simulink library "escontroller_lib"  (R2024a)
settings: Solver=VariableStepAuto  StartTime=0.0  StopTime=10.0  RelTol=1e-3
undefined symbols (not defined in the file): DiscIntNeverNeededParam, theta0
settings Model: Creator=tn212  LastModifiedBy=tn212

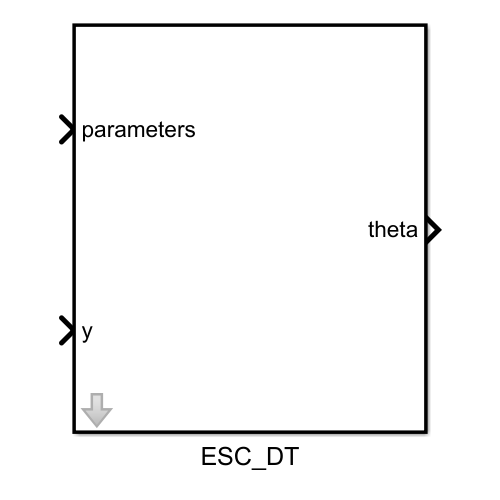
[thumbnail: Simulink's stored preview of the top-level diagram]
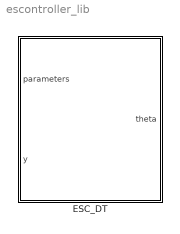
== system escontroller_lib ==
  ESC_DT : Subsystem  TreatAsAtomicUnit=on  mask{offset_sinwave_modulation=0, offset_sinwave_demodulation=0}
      mask prompts: offset_sinwave_modulation "Modulation Sine Wave Offset"; offset_sinwave_demodulation "Demodulation Sine Wave Offset"

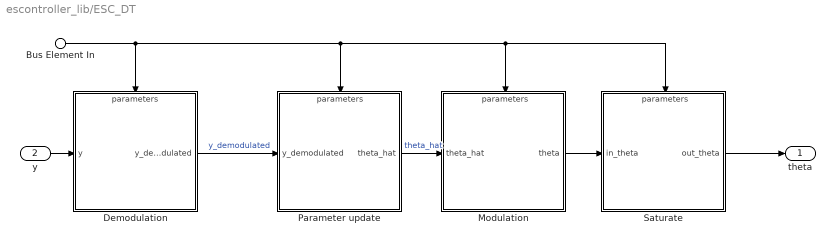
== system escontroller_lib/ESC_DT ==
  Bus Element In : Inport  PortName=parameters
  y : Inport  Port=2
  Demodulation : Subsystem
      settings: PortSchema="{\"entries\":[{\"content\":{\"sides\":[{\"content\":{\"connectorIds\":[\"In1\"]},\"type\":\"ConnectorPlacement.EquallySpacedRectSide\",\"uuid\":\"9be20e08-1b04-4097-90e8-af3e7d9708a2\"},{\"content\":{\"connectorIds\":[\"Out1\"],\"side\":\"RIGHT\"},\"type\":\"ConnectorPlacement.EquallySpacedRectSide\",\"uuid\":\"f95c4cce-30aa-41a8-9527-7dbc7585a088\"},{\"content\":{\"connectorIds\":[\"In2\"],\"side\":\"TOP\"},\"type\":\"ConnectorPlacement.EquallySpacedRectSide\",\"uuid\":\"f76abcb4-2537-40d6-8bec-356143dfe4be\"}]},\"type\":\"ConnectorPlacement.EquallySpacedConnector\",\"uuid\":\"d9c63798-3d6c-4302-a506-66d2b025211e\"}],\"packageUris\":[\"http://schema.mathworks.com/mf0/Connector/R2020b\"],\"version\":\"1.0\"}"
  Modulation : Subsystem
      settings: PortSchema="{\"entries\":[{\"content\":{\"sides\":[{\"content\":{\"connectorIds\":[\"In1\"]},\"type\":\"ConnectorPlacement.EquallySpacedRectSide\",\"uuid\":\"9be20e08-1b04-4097-90e8-af3e7d9708a2\"},{\"content\":{\"connectorIds\":[\"Out1\"],\"side\":\"RIGHT\"},\"type\":\"ConnectorPlacement.EquallySpacedRectSide\",\"uuid\":\"f95c4cce-30aa-41a8-9527-7dbc7585a088\"},{\"content\":{\"connectorIds\":[\"In2\"],\"side\":\"TOP\"},\"type\":\"ConnectorPlacement.EquallySpacedRectSide\",\"uuid\":\"f76abcb4-2537-40d6-8bec-356143dfe4be\"}]},\"type\":\"ConnectorPlacement.EquallySpacedConnector\",\"uuid\":\"d9c63798-3d6c-4302-a506-66d2b025211e\"}],\"packageUris\":[\"http://schema.mathworks.com/mf0/Connector/R2020b\"],\"version\":\"1.0\"}"
  Parameter update : Subsystem
      settings: PortSchema="{\"entries\":[{\"content\":{\"sides\":[{\"content\":{\"connectorIds\":[\"In1\"]},\"type\":\"ConnectorPlacement.EquallySpacedRectSide\",\"uuid\":\"9be20e08-1b04-4097-90e8-af3e7d9708a2\"},{\"content\":{\"connectorIds\":[\"Out1\"],\"side\":\"RIGHT\"},\"type\":\"ConnectorPlacement.EquallySpacedRectSide\",\"uuid\":\"f95c4cce-30aa-41a8-9527-7dbc7585a088\"},{\"content\":{\"connectorIds\":[\"In2\"],\"side\":\"TOP\"},\"type\":\"ConnectorPlacement.EquallySpacedRectSide\",\"uuid\":\"f76abcb4-2537-40d6-8bec-356143dfe4be\"}]},\"type\":\"ConnectorPlacement.EquallySpacedConnector\",\"uuid\":\"d9c63798-3d6c-4302-a506-66d2b025211e\"}],\"packageUris\":[\"http://schema.mathworks.com/mf0/Connector/R2020b\"],\"version\":\"1.0\"}"
  Saturate : Subsystem
      settings: PortSchema="{\"entries\":[{\"content\":{\"sides\":[{\"content\":{\"connectorIds\":[\"In1\"]},\"type\":\"ConnectorPlacement.EquallySpacedRectSide\",\"uuid\":\"9be20e08-1b04-4097-90e8-af3e7d9708a2\"},{\"content\":{\"connectorIds\":[\"Out1\"],\"side\":\"RIGHT\"},\"type\":\"ConnectorPlacement.EquallySpacedRectSide\",\"uuid\":\"f95c4cce-30aa-41a8-9527-7dbc7585a088\"},{\"content\":{\"connectorIds\":[\"In2\"],\"side\":\"TOP\"},\"type\":\"ConnectorPlacement.EquallySpacedRectSide\",\"uuid\":\"f76abcb4-2537-40d6-8bec-356143dfe4be\"}]},\"type\":\"ConnectorPlacement.EquallySpacedConnector\",\"uuid\":\"d9c63798-3d6c-4302-a506-66d2b025211e\"}],\"packageUris\":[\"http://schema.mathworks.com/mf0/Connector/R2020b\"],\"version\":\"1.0\"}"
  theta : Outport
  wires:
  Bus Element In/1 -> Demodulation/2(parameters), Parameter update/2(parameters), Saturate/2(parameters), Modulation/2(parameters)
  Saturate/1(out_theta) -> theta/1
  Modulation/1(theta) -> Saturate/1(in_theta)
  Demodulation/1(y_demodulated) -> Parameter update/1(y_demodulated)  "y_demodulated"
  Parameter update/1(theta_hat) -> Modulation/1(theta_hat)  "theta_hat"
  y/1 -> Demodulation/1(y)

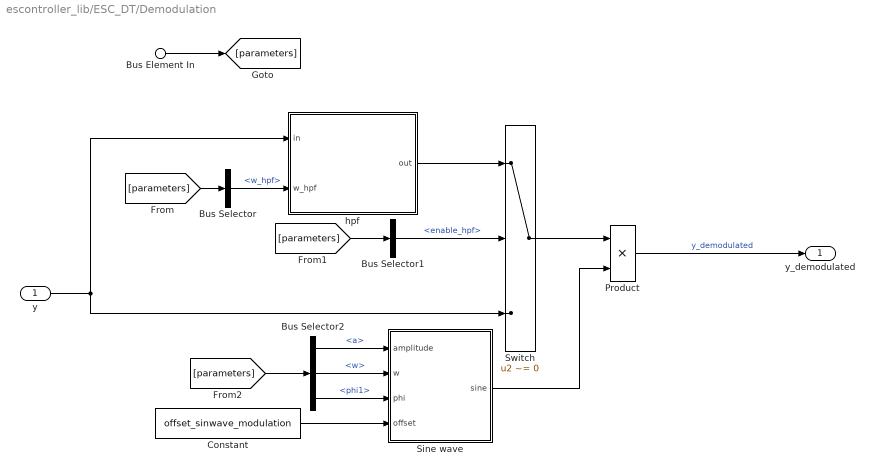
== system escontroller_lib/ESC_DT/Demodulation ==
  y : Inport
  Bus Element In : Inport  Port=2  PortName=parameters
  Bus Selector : BusSelector  OutputSignals=w_hpf
  Bus Selector1 : BusSelector  OutputSignals=enable_hpf
  Bus Selector2 : BusSelector  OutputSignals=a,w,phi1
  Constant : Constant  Value=offset_sinwave_modulation
  Product : Product
  Sine wave : Subsystem
  Switch : Switch  Criteria=u2 ~= 0  SaturateOnIntegerOverflow=off  InputSameDT=off
  hpf : Subsystem
  y_demodulated : Outport
  wires:
  Constant/1 -> Sine wave/4(offset)
  Bus Selector2/3 -> Sine wave/3(phi)  "<phi1>"
  Bus Selector2/2 -> Sine wave/2(w)  "<w>"
  Bus Selector2/1 -> Sine wave/1(amplitude)  "<a>"
  [parameters] -> Bus Selector2/1
  Bus Selector1/1 -> Switch/2  "<enable_hpf>"
  [parameters] -> Bus Selector1/1
  [parameters] -> Bus Selector/1
  Bus Element In/1 -> [parameters]
  Bus Selector/1 -> hpf/2(w_hpf)  "<w_hpf>"
  y/1 -> Switch/3, hpf/1(in)
  Switch/1 -> Product/1
  Product/1 -> y_demodulated/1  "y_demodulated"
  hpf/1(out) -> Switch/1
  Sine wave/1(sine) -> Product/2

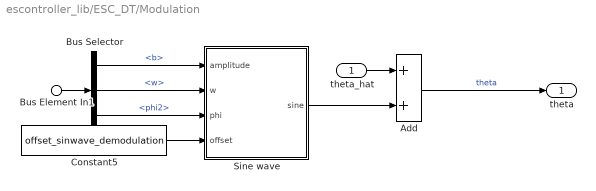
== system escontroller_lib/ESC_DT/Modulation ==
  theta_hat : Inport
  Bus Element In1 : Inport  Port=2  PortName=parameters
  Add : Sum
  Bus Selector : BusSelector  OutputSignals=b,w,phi2
  Constant5 : Constant  Value=offset_sinwave_demodulation
  Sine wave : Subsystem
  theta : Outport
  wires:
  Bus Element In1/1 -> Bus Selector/1
  Bus Selector/2 -> Sine wave/2(w)  "<w>"
  Bus Selector/1 -> Sine wave/1(amplitude)  "<b>"
  Bus Selector/3 -> Sine wave/3(phi)  "<phi2>"
  Constant5/1 -> Sine wave/4(offset)
  theta_hat/1 -> Add/1
  Add/1 -> theta/1  "theta"
  Sine wave/1(sine) -> Add/2

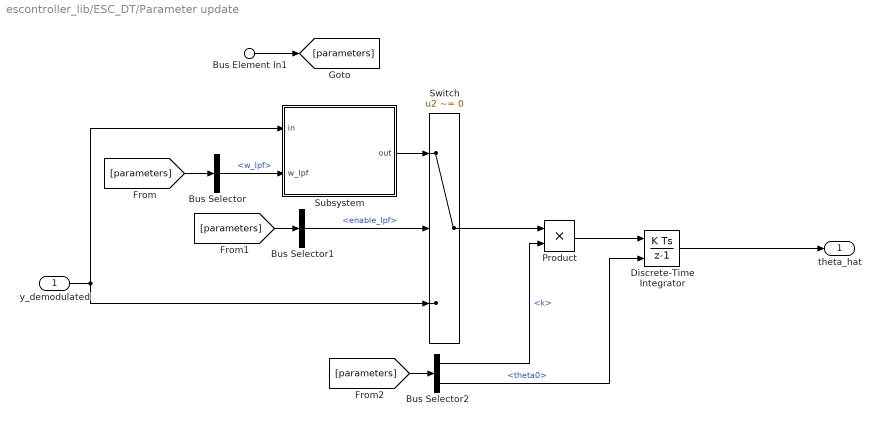
== system escontroller_lib/ESC_DT/Parameter update ==
  y_demodulated : Inport
  Bus Element In1 : Inport  Port=2  PortName=parameters
  Bus Selector : BusSelector  OutputSignals=w_lpf
  Bus Selector1 : BusSelector  OutputSignals=enable_lpf
  Bus Selector2 : BusSelector  OutputSignals=k,theta0
  Discrete-Time Integrator : DiscreteIntegrator  InitialConditionSource=external  InitialCondition=theta0  SampleTime=-1  ICPrevOutput=DiscIntNeverNeededParam  ICPrevScaledInput=DiscIntNeverNeededParam
  Product : Product
  Subsystem : Subsystem
  Switch : Switch  Criteria=u2 ~= 0  SaturateOnIntegerOverflow=off  InputSameDT=off
  theta_hat : Outport
  wires:
  [parameters] -> Bus Selector2/1
  [parameters] -> Bus Selector1/1
  [parameters] -> Bus Selector/1
  Bus Element In1/1 -> [parameters]
  Bus Selector2/2 -> Discrete-Time Integrator/2  "<theta0>"
  Bus Selector2/1 -> Product/2  "<k>"
  Switch/1 -> Product/1
  y_demodulated/1 -> Subsystem/1(in), Switch/3
  Bus Selector1/1 -> Switch/2  "<enable_lpf>"
  Discrete-Time Integrator/1 -> theta_hat/1
  Product/1 -> Discrete-Time Integrator/1
  Subsystem/1(out) -> Switch/1
  Bus Selector/1 -> Subsystem/2(w_lpf)  "<w_lpf>"

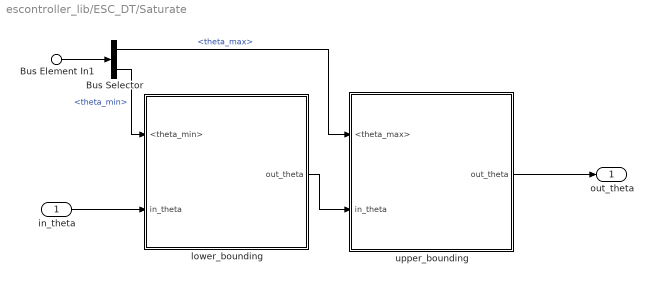
== system escontroller_lib/ESC_DT/Saturate ==
  in_theta : Inport
  Bus Element In1 : Inport  Port=2  PortName=parameters
  Bus Selector : BusSelector  OutputSignals=theta_max,theta_min
  lower_bounding : Subsystem
  upper_bounding : Subsystem
  out_theta : Outport
  wires:
  Bus Element In1/1 -> Bus Selector/1
  Bus Selector/2 -> lower_bounding/1(<theta_min>)  "<theta_min>"
  in_theta/1 -> lower_bounding/2(in_theta)
  Bus Selector/1 -> upper_bounding/1(<theta_max>)  "<theta_max>"
  lower_bounding/1(out_theta) -> upper_bounding/2(in_theta)
  upper_bounding/1(out_theta) -> out_theta/1

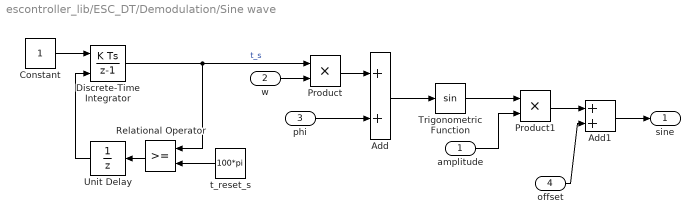
== system escontroller_lib/ESC_DT/Demodulation/Sine wave ==
  amplitude : Inport
  w : Inport  Port=2
  phi : Inport  Port=3
  offset : Inport  Port=4
  Add : Sum
  Add1 : Sum
  Constant : Constant
  Discrete-Time Integrator : DiscreteIntegrator  ExternalReset=rising  SampleTime=-1  ICPrevOutput=DiscIntNeverNeededParam  ICPrevScaledInput=DiscIntNeverNeededParam
  Product : Product
  Product1 : Product
  Relational Operator : RelationalOperator  OutDataTypeStr=boolean  RndMeth=Simplest  InputSameDT=off
  Trigonometric Function : Trigonometry
  Unit Delay : UnitDelay  SampleTime=-1  HasFrameUpgradeWarning=on
  t_reset_s : Constant  Value=100*pi
  sine : Outport
  wires:
  Constant/1 -> Discrete-Time Integrator/1
  Discrete-Time Integrator/1 -> Relational Operator/1, Product/1  "t_s"
  Product/1 -> Add/1
  phi/1 -> Add/2
  Add/1 -> Trigonometric Function/1
  t_reset_s/1 -> Relational Operator/2
  Relational Operator/1 -> Unit Delay/1
  Unit Delay/1 -> Discrete-Time Integrator/2
  w/1 -> Product/2
  Trigonometric Function/1 -> Product1/1
  amplitude/1 -> Product1/2
  Product1/1 -> Add1/1
  offset/1 -> Add1/2
  Add1/1 -> sine/1

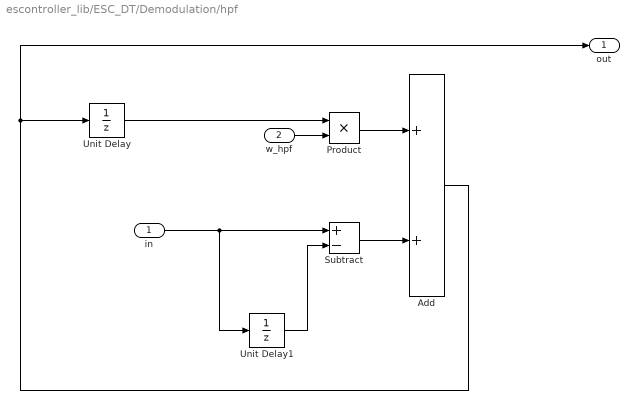
== system escontroller_lib/ESC_DT/Demodulation/hpf ==
  in : Inport
  w_hpf : Inport  Port=2
  Add : Sum
  Product : Product
  Subtract : Sum  Inputs=+-
  Unit Delay : UnitDelay  SampleTime=-1  HasFrameUpgradeWarning=on
  Unit Delay1 : UnitDelay  SampleTime=-1  HasFrameUpgradeWarning=on
  out : Outport
  wires:
  in/1 -> Unit Delay1/1, Subtract/1
  Unit Delay/1 -> Product/1
  Product/1 -> Add/1
  Unit Delay1/1 -> Subtract/2
  Subtract/1 -> Add/2
  Add/1 -> out/1, Unit Delay/1
  w_hpf/1 -> Product/2

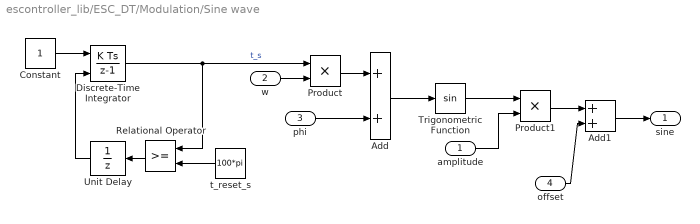
== system escontroller_lib/ESC_DT/Modulation/Sine wave ==
  amplitude : Inport
  w : Inport  Port=2
  phi : Inport  Port=3
  offset : Inport  Port=4
  Add : Sum
  Add1 : Sum
  Constant : Constant
  Discrete-Time Integrator : DiscreteIntegrator  ExternalReset=rising  SampleTime=-1  ICPrevOutput=DiscIntNeverNeededParam  ICPrevScaledInput=DiscIntNeverNeededParam
  Product : Product
  Product1 : Product
  Relational Operator : RelationalOperator  OutDataTypeStr=boolean  RndMeth=Simplest  InputSameDT=off
  Trigonometric Function : Trigonometry
  Unit Delay : UnitDelay  SampleTime=-1  HasFrameUpgradeWarning=on
  t_reset_s : Constant  Value=100*pi
  sine : Outport
  wires:
  Constant/1 -> Discrete-Time Integrator/1
  Discrete-Time Integrator/1 -> Relational Operator/1, Product/1  "t_s"
  Product/1 -> Add/1
  phi/1 -> Add/2
  Add/1 -> Trigonometric Function/1
  t_reset_s/1 -> Relational Operator/2
  Relational Operator/1 -> Unit Delay/1
  Unit Delay/1 -> Discrete-Time Integrator/2
  w/1 -> Product/2
  Trigonometric Function/1 -> Product1/1
  amplitude/1 -> Product1/2
  Product1/1 -> Add1/1
  offset/1 -> Add1/2
  Add1/1 -> sine/1

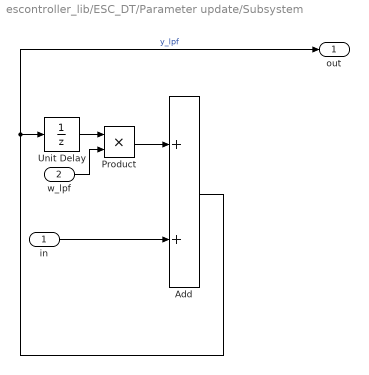
== system escontroller_lib/ESC_DT/Parameter update/Subsystem ==
  in : Inport
  w_lpf : Inport  Port=2
  Add : Sum
  Product : Product
  Unit Delay : UnitDelay  SampleTime=-1  HasFrameUpgradeWarning=on
  out : Outport
  wires:
  Add/1 -> out/1, Unit Delay/1  "y_lpf"
  in/1 -> Add/2
  Unit Delay/1 -> Product/1
  w_lpf/1 -> Product/2
  Product/1 -> Add/1

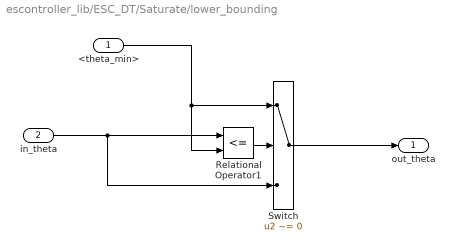
== system escontroller_lib/ESC_DT/Saturate/lower_bounding ==
  <theta_min> : Inport
  in_theta : Inport  Port=2
  Relational Operator1 : RelationalOperator  Operator=<=  OutDataTypeStr=boolean  RndMeth=Simplest  InputSameDT=off
  Switch : Switch  Criteria=u2 ~= 0  SaturateOnIntegerOverflow=off  InputSameDT=off
  out_theta : Outport
  wires:
  <theta_min>/1 -> Switch/1, Relational Operator1/2
  in_theta/1 -> Relational Operator1/1, Switch/3
  Relational Operator1/1 -> Switch/2
  Switch/1 -> out_theta/1

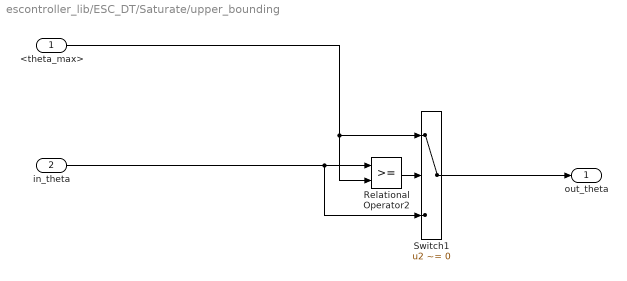
== system escontroller_lib/ESC_DT/Saturate/upper_bounding ==
  <theta_max> : Inport
  in_theta : Inport  Port=2
  Relational Operator2 : RelationalOperator  OutDataTypeStr=boolean  RndMeth=Simplest  InputSameDT=off
  Switch1 : Switch  Criteria=u2 ~= 0  SaturateOnIntegerOverflow=off  InputSameDT=off
  out_theta : Outport
  wires:
  <theta_max>/1 -> Switch1/1, Relational Operator2/2
  in_theta/1 -> Switch1/3, Relational Operator2/1
  Switch1/1 -> out_theta/1
  Relational Operator2/1 -> Switch1/2
